simulink library "Swerve_Drive_lib"  (R2023a)
settings: Solver=VariableStepAuto  StartTime=0.0  StopTime=10.0  RelTol=1e-3
undefined symbols (not defined in the file): t_sample
libraries: slpidlib x2, embmathops x2, Rotation2D x2, simulink x1
settings Model: Creator=FIRSTMentor  LastModifiedBy=FIRSTMentor

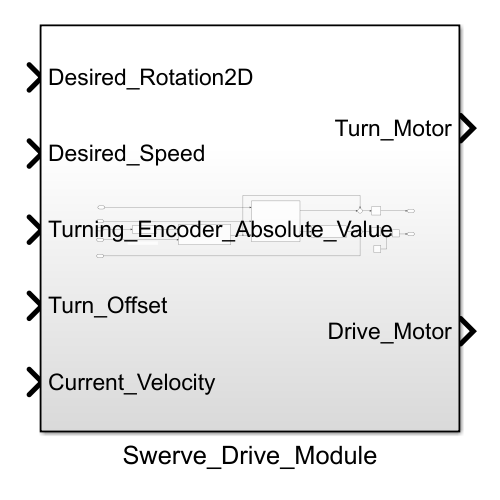
[thumbnail: Simulink's stored preview of the top-level diagram]
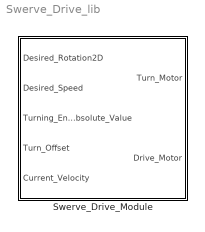
== system Swerve_Drive_lib ==
  Swerve_Drive_Module : Subsystem

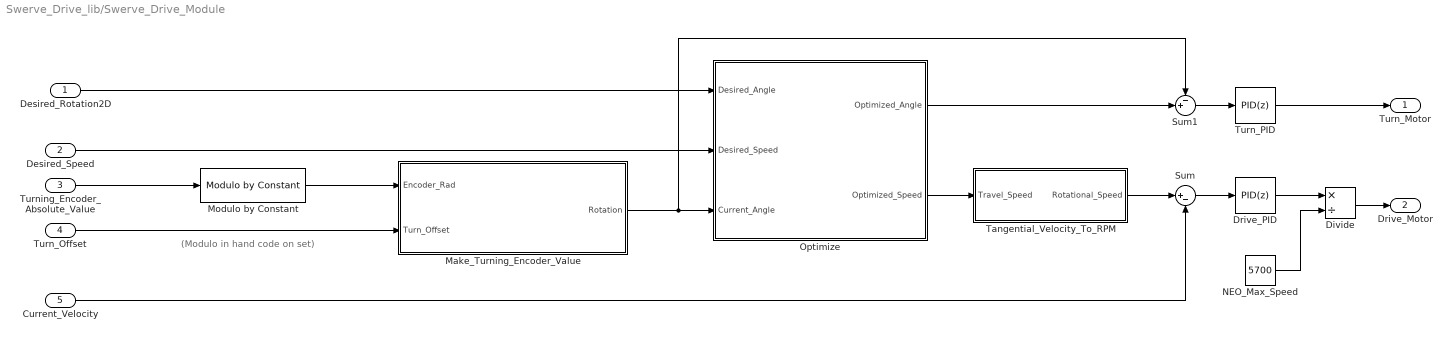
== system Swerve_Drive_lib/Swerve_Drive_Module ==
  note: (Modulo in hand code on set)
  Desired_Rotation2D : Inport  OutDataTypeStr=double  Unit=rad
  Desired_Speed : Inport  Port=2  OutDataTypeStr=double  Unit=m/s
  Turning_Encoder_Absolute_Value : Inport  Port=3  OutDataTypeStr=double  Unit=rev
  Turn_Offset : Inport  Port=4  OutDataTypeStr=double  Unit=rev
  Current_Velocity : Inport  Port=5  OutDataTypeStr=double  Unit=rpm
  Divide : Product  Inputs=*/
  Drive_PID : slpidlib/PID Controller  Controller=PID  Form=Parallel  TimeDomain=Discrete-time  UseExternalTs=off  SampleTime=t_sample  IntegratorMethod=Forward Euler  FilterMethod=Forward Euler  ControllerParametersSource=internal  P=1  I=1  UseKiTs=off  D=0  N=100  UseFilter=on  TunerSelectOption=Transfer Function Based (PID Tuner App)  InitialConditionSource=internal  InitialConditionForIntegrator=0  InitialConditionForFilter=0  DifferentiatorICPrevScaledInput=0  ExternalReset=none  TrackingMode=off  Kt=1  LimitOutput=off  SatLimitsSource=internal  UpperSaturationLimit=inf  LowerSaturationLimit=-inf  LinearizeAsGain=on  AntiWindupMode=none  Kb=1  LimitIntegrator=off  UpperIntegratorSaturationLimit=inf  LowerIntegratorSaturationLimit=-inf  POutMin=[]  POutMax=[]  IOutMin=[]  IOutMax=[]  DOutMin=[]  DOutMax=[]  NOutMin=[]  NOutMax=[]  SumOutMin=[]  SumOutMax=[]  SaturationOutMin=[]  SaturationOutMax=[]  PParamMin=[]  PParamMax=[]  IParamMin=[]  IParamMax=[]  DParamMin=[]  DParamMax=[]  NParamMin=[]  NParamMax=[]  KbParamMin=[]  KbParamMax=[]  KtParamMin=[]  KtParamMax=[]  KbOutMin=[]  KbOutMax=[]  KtOutMin=[]  KtOutMax=[]  IntegratorOutMin=[]  IntegratorOutMax=[]  FilterOutMin=[]  FilterOutMax=[]  SumI1OutMin=[]  SumI1OutMax=[]  SumI2OutMin=[]  SumI2OutMax=[]  SumI3OutMin=[]  SumI3OutMax=[]  SumI4OutMin=[]  SumI4OutMax=[]  SumDOutMin=[]  SumDOutMax=[]  DifferentiatorOutMin=[]  DifferentiatorOutMax=[]  FilterDiffOutCoefMin=[]  FilterDiffOutCoefMax=[]  ReciprocalOutMin=[]  ReciprocalOutMax=[]  SumDenOutMin=[]  SumDenOutMax=[]  SumNumOutMin=[]  SumNumOutMax=[]  DivideOutMin=[]  DivideOutMax=[]  UdiffTsProdOutMin=[]  UdiffTsProdOutMax=[]  NTsProdOutMin=[]  NTsProdOutMax=[]  UintegralTsProdOutMin=[]  UintegralTsProdOutMax=[]  UngainTsProdOutMin=[]  UngainTsProdOutMax=[]  ClampingZeroOutDataTypeStr=Inherit: Inherit via back propagation  ClampingZeroOutMin=[]  ClampingZeroOutMax=[]  FilterDenConstantOutDataTypeStr=Inherit: Inherit via back propagation  FilterDenConstantOutMin=[]  FilterDenConstantOutMax=[]  PCopyOutDataTypeStr=Inherit: Inherit via back propagation  PCopyOutMin=[]  PCopyOutMax=[]  NCopyOutDataTypeStr=Inherit: Inherit via back propagation  NCopyOutMin=[]  NCopyOutMax=[]  IntegratorContinuousStateAttributes=''  IntegratorStateMustResolveToSignalObject=off  IntegratorRTWStateStorageClass=Auto  FilterContinuousStateAttributes=''  FilterStateMustResolveToSignalObject=off  FilterRTWStateStorageClass=Auto  ParallelPVariant=InternalParameters  IdealPVariant=Disabled  IVariant=InternalParameters  DVariant=InternalParameters  IntegratorVariant=Discrete  SatVariant=Disabled  AWVariant=Passthrough  PCopyVariant=Disabled  TRVariant=Disabled  FdbkBlocksVariant=Forward  IdealPFdbkVariant=Disabled  SatFdbkVariant=Disabled  DerivativeFilterVariant=ForwardEulerFilter  NVariant=InternalParameters  NCopyVariant=Disabled  FilterICVariant=InternalICsFilter  IntegratorICVariant=InternalICs  ExternalResetVariant=Disabled  TRSumVariant=Passthrough  SumFdbkVariant=Disabled  SumVariant=Sum_PID  TsampFilterVariant=InternalTs  TsampNgainVariant=Passthrough  TsampIntegralVariant=Disabled_SignalSpec  ExternalSaturationOutDataTypeStr=Inherit: Same as second input
  Make_Turning_Encoder_Value : Subsystem
  Modulo by Constant : embmathops/Modulo by Constant  Denominator=1  SimulateUsing=Code generation
      settings: LibrarySourceBlock=embeddedMathLib/Modulo by Constant
  NEO_Max_Speed : Constant  Value=5700
  Optimize : Subsystem
  Sum : Sum  Inputs=|+-
  Sum1 : Sum  Inputs=-+|
  Tangential_Velocity_To_RPM : Subsystem
  Turn_PID : slpidlib/PID Controller  Controller=PID  Form=Parallel  TimeDomain=Discrete-time  UseExternalTs=off  SampleTime=t_sample  IntegratorMethod=Forward Euler  FilterMethod=Forward Euler  ControllerParametersSource=internal  P=1  I=1  UseKiTs=off  D=0  N=100  UseFilter=on  TunerSelectOption=Transfer Function Based (PID Tuner App)  InitialConditionSource=internal  InitialConditionForIntegrator=0  InitialConditionForFilter=0  DifferentiatorICPrevScaledInput=0  ExternalReset=none  TrackingMode=off  Kt=1  LimitOutput=off  SatLimitsSource=internal  UpperSaturationLimit=inf  LowerSaturationLimit=-inf  LinearizeAsGain=on  AntiWindupMode=none  Kb=1  LimitIntegrator=off  UpperIntegratorSaturationLimit=inf  LowerIntegratorSaturationLimit=-inf  POutMin=[]  POutMax=[]  IOutMin=[]  IOutMax=[]  DOutMin=[]  DOutMax=[]  NOutMin=[]  NOutMax=[]  SumOutMin=[]  SumOutMax=[]  SaturationOutMin=[]  SaturationOutMax=[]  PParamMin=[]  PParamMax=[]  IParamMin=[]  IParamMax=[]  DParamMin=[]  DParamMax=[]  NParamMin=[]  NParamMax=[]  KbParamMin=[]  KbParamMax=[]  KtParamMin=[]  KtParamMax=[]  KbOutMin=[]  KbOutMax=[]  KtOutMin=[]  KtOutMax=[]  IntegratorOutMin=[]  IntegratorOutMax=[]  FilterOutMin=[]  FilterOutMax=[]  SumI1OutMin=[]  SumI1OutMax=[]  SumI2OutMin=[]  SumI2OutMax=[]  SumI3OutMin=[]  SumI3OutMax=[]  SumI4OutMin=[]  SumI4OutMax=[]  SumDOutMin=[]  SumDOutMax=[]  DifferentiatorOutMin=[]  DifferentiatorOutMax=[]  FilterDiffOutCoefMin=[]  FilterDiffOutCoefMax=[]  ReciprocalOutMin=[]  ReciprocalOutMax=[]  SumDenOutMin=[]  SumDenOutMax=[]  SumNumOutMin=[]  SumNumOutMax=[]  DivideOutMin=[]  DivideOutMax=[]  UdiffTsProdOutMin=[]  UdiffTsProdOutMax=[]  NTsProdOutMin=[]  NTsProdOutMax=[]  UintegralTsProdOutMin=[]  UintegralTsProdOutMax=[]  UngainTsProdOutMin=[]  UngainTsProdOutMax=[]  ClampingZeroOutDataTypeStr=Inherit: Inherit via back propagation  ClampingZeroOutMin=[]  ClampingZeroOutMax=[]  FilterDenConstantOutDataTypeStr=Inherit: Inherit via back propagation  FilterDenConstantOutMin=[]  FilterDenConstantOutMax=[]  PCopyOutDataTypeStr=Inherit: Inherit via back propagation  PCopyOutMin=[]  PCopyOutMax=[]  NCopyOutDataTypeStr=Inherit: Inherit via back propagation  NCopyOutMin=[]  NCopyOutMax=[]  IntegratorContinuousStateAttributes=''  IntegratorStateMustResolveToSignalObject=off  IntegratorRTWStateStorageClass=Auto  FilterContinuousStateAttributes=''  FilterStateMustResolveToSignalObject=off  FilterRTWStateStorageClass=Auto  ParallelPVariant=InternalParameters  IdealPVariant=Disabled  IVariant=InternalParameters  DVariant=InternalParameters  IntegratorVariant=Discrete  SatVariant=Disabled  AWVariant=Passthrough  PCopyVariant=Disabled  TRVariant=Disabled  FdbkBlocksVariant=Forward  IdealPFdbkVariant=Disabled  SatFdbkVariant=Disabled  DerivativeFilterVariant=ForwardEulerFilter  NVariant=InternalParameters  NCopyVariant=Disabled  FilterICVariant=InternalICsFilter  IntegratorICVariant=InternalICs  ExternalResetVariant=Disabled  TRSumVariant=Passthrough  SumFdbkVariant=Disabled  SumVariant=Sum_PID  TsampFilterVariant=InternalTs  TsampNgainVariant=Passthrough  TsampIntegralVariant=Disabled_SignalSpec  ExternalSaturationOutDataTypeStr=Inherit: Same as second input
  Turn_Motor : Outport  OutDataTypeStr=double  Unit=1
  Drive_Motor : Outport  Port=2  OutDataTypeStr=double  Unit=1
  wires:
  Current_Velocity/1 -> Sum/2
  Desired_Rotation2D/1 -> Optimize/1(Desired_Angle)
  Modulo by Constant/1 -> Make_Turning_Encoder_Value/1(Encoder_Rad)
  NEO_Max_Speed/1 -> Divide/2
  Sum1/1 -> Turn_PID/1
  Desired_Speed/1 -> Optimize/2(Desired_Speed)
  Optimize/2(Optimized_Speed) -> Tangential_Velocity_To_RPM/1(Travel_Speed)
  Divide/1 -> Drive_Motor/1
  Tangential_Velocity_To_RPM/1(Rotational_Speed) -> Sum/1
  Turning_Encoder_Absolute_Value/1 -> Modulo by Constant/1
  Optimize/1(Optimized_Angle) -> Sum1/2
  Make_Turning_Encoder_Value/1(Rotation) -> Optimize/3(Current_Angle), Sum1/1
  Turn_PID/1 -> Turn_Motor/1
  Drive_PID/1 -> Divide/1
  Sum/1 -> Drive_PID/1
  Turn_Offset/1 -> Make_Turning_Encoder_Value/2(Turn_Offset)

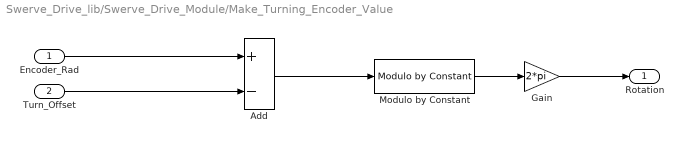
== system Swerve_Drive_lib/Swerve_Drive_Module/Make_Turning_Encoder_Value ==
  Encoder_Rad : Inport  OutDataTypeStr=double  Unit=rev
  Turn_Offset : Inport  Port=2  OutDataTypeStr=double  Unit=rev
  Add : Sum  Inputs=+-
  Gain : Gain  Gain=2*pi
  Modulo by Constant : embmathops/Modulo by Constant  Denominator=1  SimulateUsing=Code generation
      settings: LibrarySourceBlock=embeddedMathLib/Modulo by Constant
  Rotation : Outport  OutDataTypeStr=double  Unit=rad
  wires:
  Modulo by Constant/1 -> Gain/1
  Add/1 -> Modulo by Constant/1
  Turn_Offset/1 -> Add/2
  Encoder_Rad/1 -> Add/1
  Gain/1 -> Rotation/1

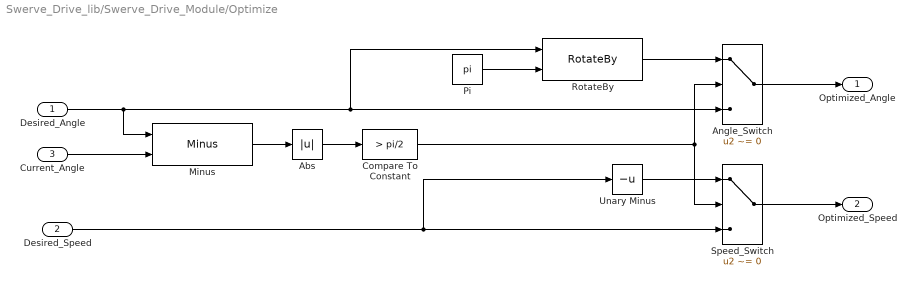
== system Swerve_Drive_lib/Swerve_Drive_Module/Optimize ==
  Desired_Angle : Inport  OutDataTypeStr=double  Unit=rad
  Desired_Speed : Inport  Port=2  OutDataTypeStr=double  Unit=m/s
  Current_Angle : Inport  Port=3  OutDataTypeStr=double  Unit=rad
  Abs : Abs  SaturateOnIntegerOverflow=off
  Angle_Switch : Switch  Criteria=u2 ~= 0  SaturateOnIntegerOverflow=off  InputSameDT=off
  Compare To Constant : simulink/Logic and Bit Operations/Compare To Constant  relop=>  const=pi/2  OutDataTypeStr=boolean
  Minus : Rotation2D/Minus  SystemSampleTime=-1  VariantActivationTime=update diagram  Latency=0  AutoFrameSizeCalculation=off
  Pi : Constant  Value=pi  OutDataTypeStr=Inherit: Inherit via back propagation
  RotateBy : Rotation2D/RotateBy  SystemSampleTime=-1  VariantActivationTime=update diagram  Latency=0  AutoFrameSizeCalculation=off
  Speed_Switch : Switch  Criteria=u2 ~= 0  SaturateOnIntegerOverflow=off  InputSameDT=off
  Unary Minus : UnaryMinus
  Optimized_Angle : Outport  OutDataTypeStr=double  Unit=rad
  Optimized_Speed : Outport  Port=2  OutDataTypeStr=double  Unit=m/s
  wires:
  Desired_Angle/1 -> RotateBy/1, Angle_Switch/3, Minus/1
  Current_Angle/1 -> Minus/2
  Minus/1 -> Abs/1
  Abs/1 -> Compare To Constant/1
  Desired_Speed/1 -> Unary Minus/1, Speed_Switch/3
  Compare To Constant/1 -> Angle_Switch/2, Speed_Switch/2
  Unary Minus/1 -> Speed_Switch/1
  Pi/1 -> RotateBy/2
  RotateBy/1 -> Angle_Switch/1
  Angle_Switch/1 -> Optimized_Angle/1
  Speed_Switch/1 -> Optimized_Speed/1

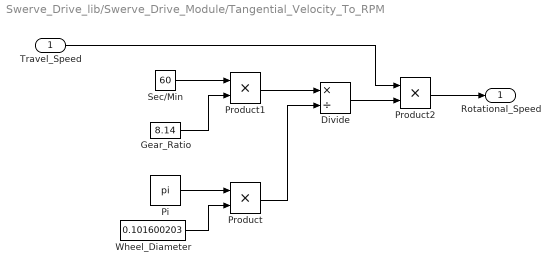
== system Swerve_Drive_lib/Swerve_Drive_Module/Tangential_Velocity_To_RPM ==
  Travel_Speed : Inport  Unit=m/s
  Divide : Product  Inputs=*/
  Gear_Ratio : Constant  Value=8.14
  Pi : Constant  Value=pi  OutDataTypeStr=Inherit: Inherit via back propagation
  Product : Product
  Product1 : Product
  Product2 : Product
  Sec/Min : Constant  Value=60
  Wheel_Diameter : Constant  Value=0.101600203
  Rotational_Speed : Outport  Unit=rpm
  wires:
  Product/1 -> Divide/2
  Pi/1 -> Product/1
  Product1/1 -> Divide/1
  Sec/Min/1 -> Product1/1
  Gear_Ratio/1 -> Product1/2
  Product2/1 -> Rotational_Speed/1
  Wheel_Diameter/1 -> Product/2
  Travel_Speed/1 -> Product2/1
  Divide/1 -> Product2/2
